simulink model "complementaryAndroidAHRS"  (R2019a)
settings: Solver=FixedStepAuto  StartTime=0.0  StopTime=40  RelTol=1e-3
InitFcn:
  | Ts=0.004
undefined symbols (not defined in the file): DiscIntNeverNeededParam
libraries: simulink_extras x8, androiduilib x6, dspstat3 x3, androidsensorlib x3
PreSaveFcn:
  | set_param(gcs, 'Location',[35 56 895 605])
settings Model: SimulationMode=external  ExtModeTrigDuration=100  Creator=The MathWorks, Inc.  LastModifiedBy=Alireza
settings DataIOCC: LimitDataPoints=on  SaveFormat=Array  ReturnWorkspaceOutputs=off
settings OptimizationCC: LifeSpan=1  MaxStackSize=64
settings DebuggingCC: UnderspecifiedInitializationDetection=Classic  MergeDetectMultiDrivingBlocksExec=none  ParameterPrecisionLossMsg=none  AllowSymbolicDim=off  SFUnexpectedBacktrackingDiag=warning  SFNoUnconditionalDefaultTransitionDiag=warning  SFExecutionAtInitializationDiag=none  ArithmeticOperatorsInVariantConditions=warning
settings HardwareCC: ProdBitPerPointer=32  ProdBitPerSizeT=32  ProdBitPerPtrDiffT=32  ProdLargestAtomicInteger=Long  ProdLargestAtomicFloat=Double  ProdWordSize=32  ProdHWDeviceType=ARM Compatible->ARM Cortex  TargetLargestAtomicInteger=Long  TargetLargestAtomicFloat=Double  TargetEndianess=LittleEndian  TargetHWDeviceType=ARM Compatible->ARM Cortex
settings ModelReferenceCC: PropagateSignalLabelsOutOfModel=off
settings SFSimCC: SimUseLocalCustomCode=off
settings RTWCC: SystemTargetFile=ert.tlc  HardwareBoard=Android Device  TLCOptions="-aInlineSetEventsForThisBaseRateFcn=TLC_FALSE -aSuppressMultiTaskScheduler=TLC_FALSE  -aRateBasedStepFcn=0"  TemplateMakefile=ert_default_tmf  GenerateReport=on  RTWVerbose=off  RTWUseLocalCustomCode=off  Toolchain=Android SDK/NDK Tools  LaunchReport=on
settings CodeAppCC: ForceParamTrailComments=on  OperatorAnnotations=on  MangleLength=10  StateflowObjectComments=on  MATLABSourceComments=on
settings ERTTargetCC: MultiwordLength=2048  ERTCustomFileBanners=off  SupportContinuousTime=on  SupportNonInlinedSFcns=on  RemoveResetFunc=off  SupportVariableSizeSignals=on  ModelStepFunctionPrototypeControlCompliant=off
settings ConfigComp: CovMetricSettings=dw  CovHtmlReporting=on  CovSaveCumulativeToWorkspaceVar=on  CovSaveSingleToWorkspaceVar=on  CovExternalEMLEnable=off  CovSFcnEnable=off

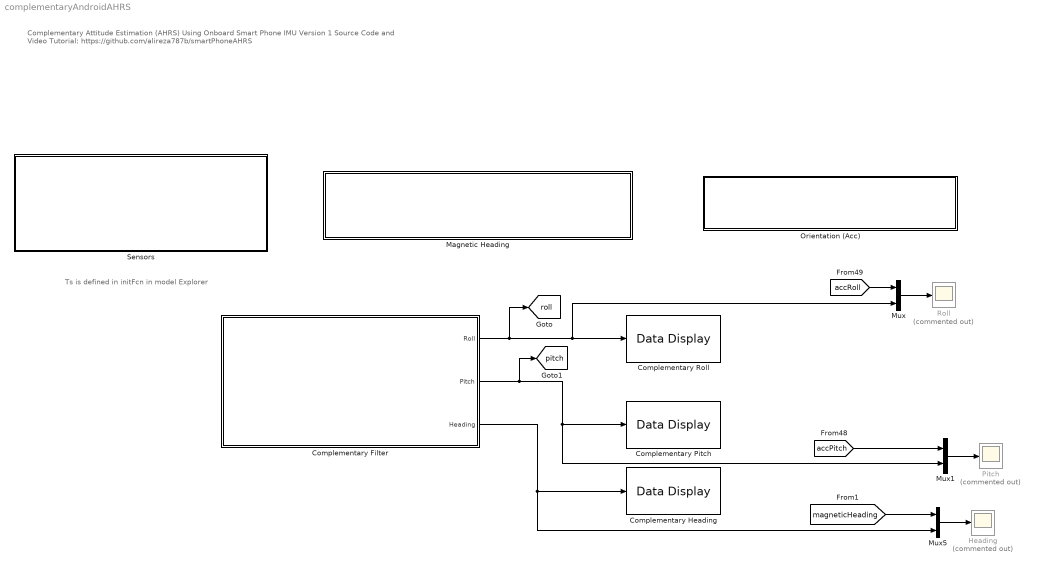
== system complementaryAndroidAHRS ==
  note: Ts is defined in initFcn in model Explorer
  note: Complementary Attitude Estimation (AHRS)
      | Using Onboard Smart Phone IMU Version 1
      | Source Code and Video Tutorial:
      | https://github.com/alireza787b/smartPhoneAHRS
  Complementary Filter : Subsystem
  Complementary Heading : androiduilib/Data Display  DataDisplayId=complementaryAndroidAHRS/Complementary_Heading  Format=Float  Precision=6  SimulateUsing=Code generation  blockPlatform=Android
      settings: SourceProductBaseCode=ANDROID
  Complementary Pitch : androiduilib/Data Display  DataDisplayId=complementaryAndroidAHRS/Complementary_Pitch  Format=Float  Precision=6  SimulateUsing=Code generation  blockPlatform=Android
      settings: SourceProductBaseCode=ANDROID
  Complementary Roll : androiduilib/Data Display  DataDisplayId=complementaryAndroidAHRS/Complementary_Roll  Format=Float  Precision=6  SimulateUsing=Code generation  blockPlatform=Android
      settings: SourceProductBaseCode=ANDROID
  Heading : Scope  Commented=on
  Magnetic Heading : Subsystem
  Mux : Mux  Inputs=2
  Mux1 : Mux  Inputs=2
  Mux5 : Mux  Inputs=2
  Orientation (Acc) : Subsystem
  Pitch : Scope  Commented=on
  Roll : Scope  Commented=on
  Sensors : Subsystem
  tag scope: pitch=global, roll=global
  wires:
  Mux/1 -> Roll/1
  Mux1/1 -> Pitch/1
  Mux5/1 -> Heading/1
  [accPitch] -> Mux1/1
  [accRoll] -> Mux/1
  Complementary Filter/1(Roll) -> Complementary Roll/1, Mux/2, [roll]
  Complementary Filter/2("Pitch ") -> Complementary Pitch/1, Mux1/2, [pitch]
  Complementary Filter/3(Heading) -> Mux5/2, Complementary Heading/1
  [magneticHeading] -> Mux5/1

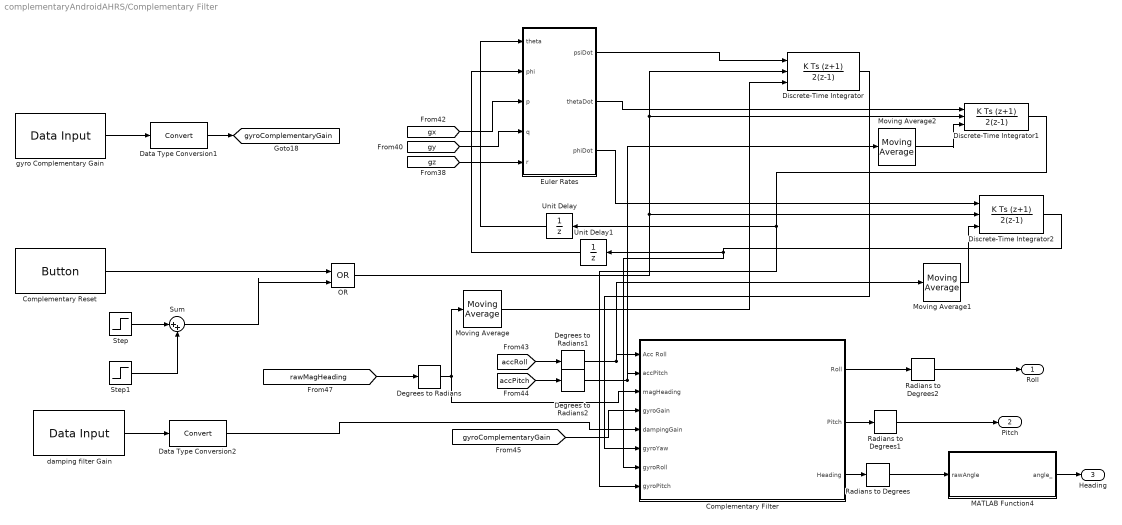
== system complementaryAndroidAHRS/Complementary Filter ==
  Complementary Filter : Subsystem
  Complementary Reset : androiduilib/Button  ButtonState=Not pressed  ButtonId=complementaryAndroidAHRS/Complementary_Filter/Complementary_Reset  State=off  SampleTime=0.1  BlockPlatform=Android
      settings: SourceProductBaseCode=ANDROID
  Data Type Conversion1 : DataTypeConversion
  Data Type Conversion2 : DataTypeConversion
  Degrees to Radians : simulink_extras/Transformations/Degrees to Radians
  Degrees to Radians1 : simulink_extras/Transformations/Degrees to Radians
  Degrees to Radians2 : simulink_extras/Transformations/Degrees to Radians
  Discrete-Time Integrator : DiscreteIntegrator  IntegratorMethod=Integration: Trapezoidal  ExternalReset=either  InitialConditionSource=external  SampleTime=-1  ICPrevOutput=DiscIntNeverNeededParam  ICPrevScaledInput=DiscIntNeverNeededParam
  Discrete-Time Integrator1 : DiscreteIntegrator  IntegratorMethod=Integration: Trapezoidal  ExternalReset=either  InitialConditionSource=external  SampleTime=-1  ICPrevOutput=DiscIntNeverNeededParam  ICPrevScaledInput=DiscIntNeverNeededParam
  Discrete-Time Integrator2 : DiscreteIntegrator  IntegratorMethod=Integration: Trapezoidal  ExternalReset=falling  InitialConditionSource=external  SampleTime=-1  ICPrevOutput=DiscIntNeverNeededParam  ICPrevScaledInput=DiscIntNeverNeededParam
  Euler Rates : Subsystem
  MATLAB Function4 : MATLAB Function  TreatAsAtomicUnit=on
  Moving Average : dspstat3/Moving Average  Method=Sliding window  ForgettingFactorPort=off  SpecifyWindowLength=on  WindowLength=4  ForgettingFactor=0.9  SimulateUsing=Code generation
  Moving Average1 : dspstat3/Moving Average  Method=Sliding window  ForgettingFactorPort=off  SpecifyWindowLength=on  WindowLength=4  ForgettingFactor=0.9  SimulateUsing=Code generation
  Moving Average2 : dspstat3/Moving Average  Method=Sliding window  ForgettingFactorPort=off  SpecifyWindowLength=on  WindowLength=4  ForgettingFactor=0.9  SimulateUsing=Code generation
  OR : Logic  Operator=OR  IconShape=distinctive  AllPortsSameDT=off  OutDataTypeStr=boolean
  Radians to Degrees : simulink_extras/Transformations/Radians to Degrees
  Radians to Degrees1 : simulink_extras/Transformations/Radians to Degrees
  Radians to Degrees2 : simulink_extras/Transformations/Radians to Degrees
  Step : Step  SampleTime=0
  Step1 : Step  Time=2  After=-1  SampleTime=0
  Sum : Sum  Inputs=|++
  Unit Delay : UnitDelay  SampleTime=-1  HasFrameUpgradeWarning=on
  Unit Delay1 : UnitDelay  SampleTime=-1  HasFrameUpgradeWarning=on
  damping filter Gain : androiduilib/Data Input  isCharVector=off  Value=0.9  CharVector=Hello World  OutputDataType=double  maxCharVectorSize=100  DataInputId=complementaryAndroidAHRS/Complementary_Filter/damping_filter_Gain  SampleTime=0.1
      settings: SourceProductBaseCode=ANDROID
  gyro Complementary Gain : androiduilib/Data Input  isCharVector=off  Value=0.78  CharVector=Hello World  OutputDataType=double  maxCharVectorSize=100  DataInputId=complementaryAndroidAHRS/Complementary_Filter/gyro_Complementary_Gain  SampleTime=0.1
      settings: SourceProductBaseCode=ANDROID
  Roll : Outport
  "Pitch " : Outport  Port=2
  Heading : Outport  Port=3
  tag scope: gyroComplementaryGain=global
  wires:
  [gy] -> Euler Rates/4(q)
  Euler Rates/3(phiDot) -> Discrete-Time Integrator2/1
  gyro Complementary Gain/1 -> Data Type Conversion1/1
  Complementary Filter/3(Heading) -> Radians to Degrees/1
  Euler Rates/1(psiDot) -> Discrete-Time Integrator/1
  Discrete-Time Integrator/1 -> Complementary Filter/6(gyroYaw)
  Unit Delay/1 -> Euler Rates/1(theta)
  Complementary Filter/1(Roll) -> Radians to Degrees2/1
  Unit Delay1/1 -> Euler Rates/2(phi)
  Degrees to Radians/1 -> Moving Average/1, Complementary Filter/3(magHeading)
  Discrete-Time Integrator1/1 -> Unit Delay/1, Complementary Filter/8(gyroPitch)
  [accRoll] -> Degrees to Radians1/1
  [gyroComplementaryGain] -> Complementary Filter/4(gyroGain)
  Discrete-Time Integrator2/1 -> Unit Delay1/1, Complementary Filter/7(gyroRoll)
  [rawMagHeading] -> Degrees to Radians/1
  [gx] -> Euler Rates/3(p)
  Euler Rates/2(thetaDot) -> Discrete-Time Integrator1/1
  [gz] -> Euler Rates/5(r)
  [accPitch] -> Degrees to Radians2/1
  Complementary Filter/2(Pitch) -> Radians to Degrees1/1
  Radians to Degrees1/1 -> "Pitch "/1
  Radians to Degrees2/1 -> Roll/1
  Radians to Degrees/1 -> MATLAB Function4/1(rawAngle)
  OR/1 -> Discrete-Time Integrator/2, Discrete-Time Integrator1/2, Discrete-Time Integrator2/2
  Moving Average/1 -> Discrete-Time Integrator/3
  Moving Average1/1 -> Discrete-Time Integrator2/3
  Moving Average2/1 -> Discrete-Time Integrator1/3
  Degrees to Radians1/1 -> Moving Average1/1, Complementary Filter/1(Acc Roll)
  Degrees to Radians2/1 -> Moving Average2/1, Complementary Filter/2(accPitch)
  MATLAB Function4/1(angle_) -> Heading/1
  Data Type Conversion1/1 -> [gyroComplementaryGain]
  Complementary Reset/1 -> OR/1
  Step/1 -> Sum/1
  Step1/1 -> Sum/2
  Sum/1 -> OR/2
  damping filter Gain/1 -> Data Type Conversion2/1
  Data Type Conversion2/1 -> Complementary Filter/5(dampingGain)

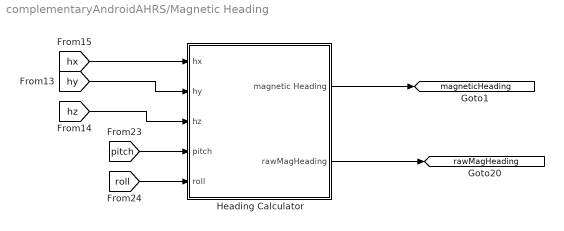
== system complementaryAndroidAHRS/Magnetic Heading ==
  Heading Calculator : Subsystem
  tag scope: magneticHeading=global, rawMagHeading=global
  wires:
  [hz] -> Heading Calculator/3(hz)
  [hy] -> Heading Calculator/2(hy)
  [hx] -> Heading Calculator/1(hx)
  [pitch] -> Heading Calculator/4(pitch)
  [roll] -> Heading Calculator/5(roll)
  Heading Calculator/2(rawMagHeading) -> [rawMagHeading]
  Heading Calculator/1(magnetic Heading) -> [magneticHeading]

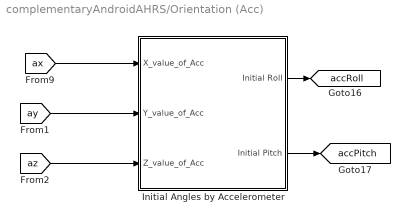
== system complementaryAndroidAHRS/Orientation (Acc) ==
  Initial Angles by Accelerometer : Subsystem
  tag scope: accPitch=global, accRoll=global
  wires:
  [ax] -> Initial Angles by Accelerometer/1(X_value_of_Acc)
  Initial Angles by Accelerometer/2(Initial Pitch) -> [accPitch]
  [ay] -> Initial Angles by Accelerometer/2(Y_value_of_Acc)
  [az] -> Initial Angles by Accelerometer/3(Z_value_of_Acc)
  Initial Angles by Accelerometer/1(Initial Roll) -> [accRoll]

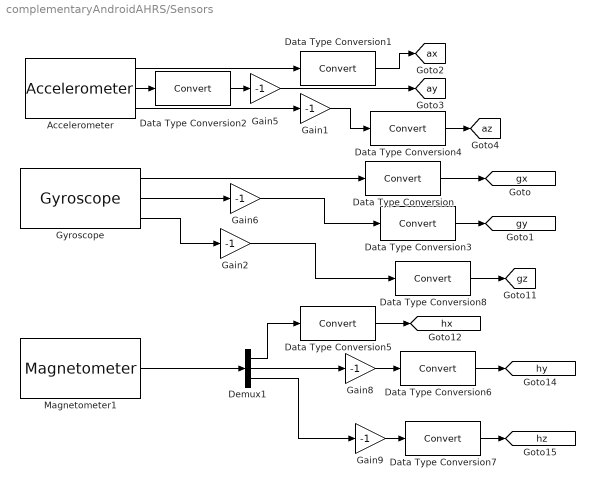
== system complementaryAndroidAHRS/Sensors ==
  Accelerometer : androidsensorlib/Accelerometer  OutputVector=off  SampleTime=Ts  BlockPlatform=Android
      settings: SourceProductBaseCode=ANDROID
  Data Type Conversion{,1..8} (9 alike) : DataTypeConversion
  Demux1 : Demux  Outputs=3
  Gain{1..2,5..6,8..9} (6 alike) : Gain  Gain=-1
  Gyroscope : androidsensorlib/Gyroscope  OutputVector=off  SampleTime=Ts  BlockPlatform=Android
      settings: SourceProductBaseCode=ANDROID
  Magnetometer1 : androidsensorlib/Magnetometer  SampleTime=0.01  SimulateUsing=Code generation
      settings: SourceProductBaseCode=ANDROID
  tag scope: ax=global, ay=global, az=global, gx=global, gy=global, gz=global, hx=global, hy=global, hz=global
  wires:
  Demux1/1 -> Data Type Conversion5/1
  Gain8/1 -> Data Type Conversion6/1
  Data Type Conversion6/1 -> [hy]
  Accelerometer/2 -> Data Type Conversion2/1
  Demux1/3 -> Gain9/1
  Data Type Conversion5/1 -> [hx]
  Gain1/1 -> Data Type Conversion4/1
  Accelerometer/3 -> Gain1/1
  Gyroscope/2 -> Gain6/1
  Data Type Conversion7/1 -> [hz]
  Gain2/1 -> Data Type Conversion8/1
  Data Type Conversion4/1 -> [az]
  Gyroscope/1 -> Data Type Conversion/1
  Data Type Conversion3/1 -> [gy]
  Gain9/1 -> Data Type Conversion7/1
  Gain5/1 -> [ay]
  Data Type Conversion/1 -> [gx]
  Magnetometer1/1 -> Demux1/1
  Gain6/1 -> Data Type Conversion3/1
  Accelerometer/1 -> Data Type Conversion1/1
  Gyroscope/3 -> Gain2/1
  Demux1/2 -> Gain8/1
  Data Type Conversion8/1 -> [gz]
  Data Type Conversion2/1 -> Gain5/1
  Data Type Conversion1/1 -> [ax]

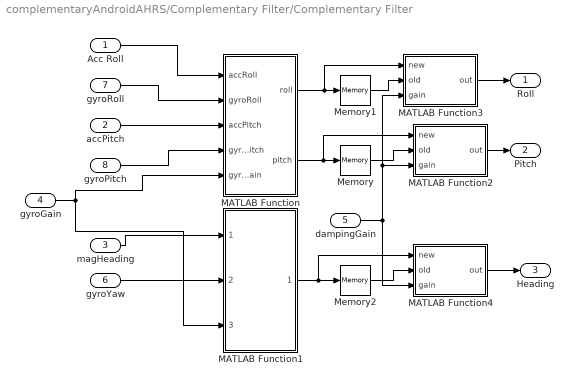
== system complementaryAndroidAHRS/Complementary Filter/Complementary Filter ==
  Acc Roll : Inport
  accPitch : Inport  Port=2
  magHeading : Inport  Port=3
  gyroGain : Inport  Port=4
  dampingGain : Inport  Port=5
  gyroYaw : Inport  Port=6
  gyroRoll : Inport  Port=7
  gyroPitch : Inport  Port=8
  MATLAB Function : MATLAB Function  TreatAsAtomicUnit=on
  MATLAB Function1 : MATLAB Function  TreatAsAtomicUnit=on
  MATLAB Function2 : MATLAB Function  TreatAsAtomicUnit=on
  MATLAB Function3 : MATLAB Function  TreatAsAtomicUnit=on
  MATLAB Function4 : MATLAB Function  TreatAsAtomicUnit=on
  Memory : Memory
  Memory1 : Memory
  Memory2 : Memory
  Roll : Outport
  Pitch : Outport  Port=2
  Heading : Outport  Port=3
  wires:
  MATLAB Function/2(pitch) -> MATLAB Function2/1(new), Memory/1
  gyroPitch/1 -> MATLAB Function/4(gyroPitch)
  accPitch/1 -> MATLAB Function/3(accPitch)
  gyroRoll/1 -> MATLAB Function/2(gyroRoll)
  Acc Roll/1 -> MATLAB Function/1(accRoll)
  gyroYaw/1 -> MATLAB Function1/2(gyroYaw)
  magHeading/1 -> MATLAB Function1/1(magHeading)
  MATLAB Function1/1(heading) -> MATLAB Function4/1(new), Memory2/1
  MATLAB Function/1(roll) -> MATLAB Function3/1(new), Memory1/1
  Memory/1 -> MATLAB Function2/2(old)
  MATLAB Function2/1(out) -> Pitch/1
  MATLAB Function3/1(out) -> Roll/1
  Memory1/1 -> MATLAB Function3/2(old)
  Memory2/1 -> MATLAB Function4/2(old)
  MATLAB Function4/1(out) -> Heading/1
  gyroGain/1 -> MATLAB Function1/3(gyroGainHeading), MATLAB Function/5(gyroGain)
  dampingGain/1 -> MATLAB Function3/3(gain), MATLAB Function2/3(gain), MATLAB Function4/3(gain)

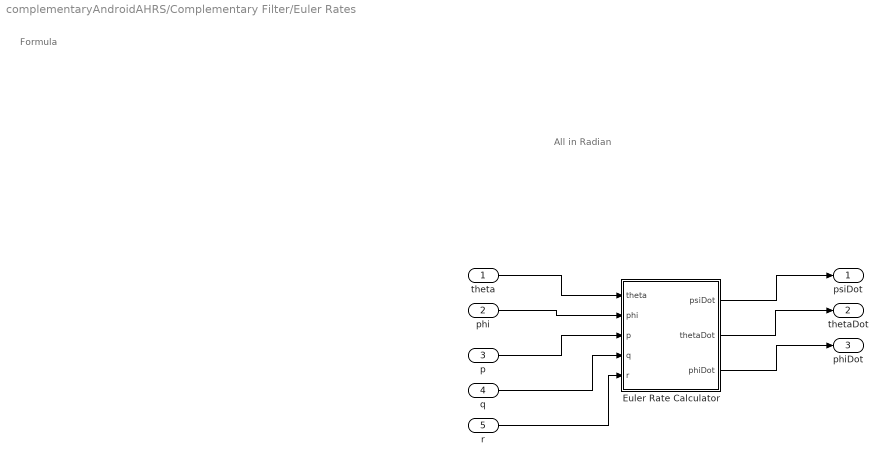
== system complementaryAndroidAHRS/Complementary Filter/Euler Rates ==
  note: All in Radian
  note: Formula
  theta : Inport
  phi : Inport  Port=2
  p : Inport  Port=3
  q : Inport  Port=4
  r : Inport  Port=5
  Euler Rate Calculator : MATLAB Function  TreatAsAtomicUnit=on
  psiDot : Outport
  thetaDot : Outport  Port=2
  phiDot : Outport  Port=3
  wires:
  phi/1 -> Euler Rate Calculator/2(phi)
  theta/1 -> Euler Rate Calculator/1(theta)
  p/1 -> Euler Rate Calculator/3(p)
  q/1 -> Euler Rate Calculator/4(q)
  r/1 -> Euler Rate Calculator/5(r)
  Euler Rate Calculator/1(psiDot) -> psiDot/1
  Euler Rate Calculator/2(thetaDot) -> thetaDot/1
  Euler Rate Calculator/3(phiDot) -> phiDot/1

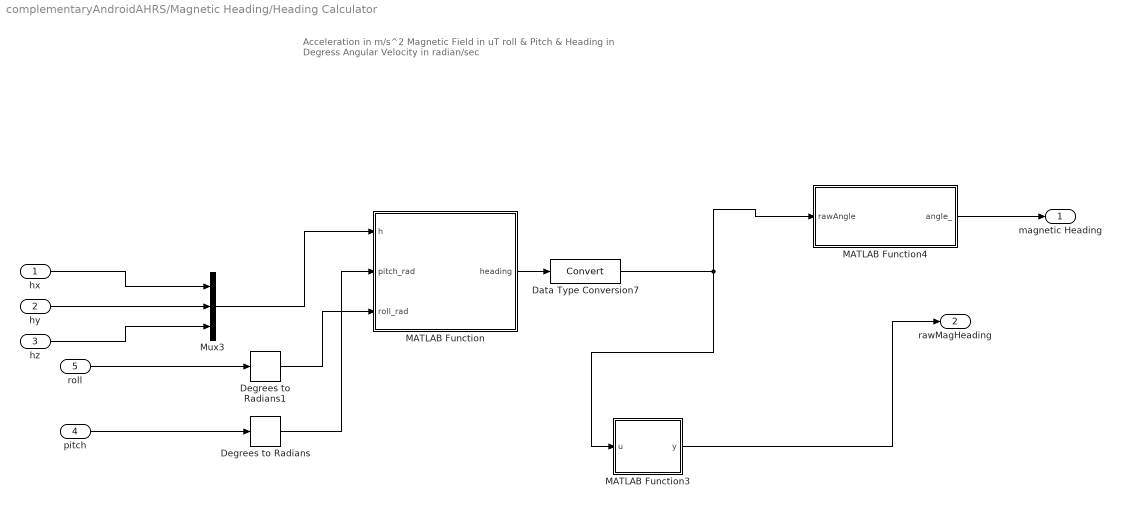
== system complementaryAndroidAHRS/Magnetic Heading/Heading Calculator ==
  note: Acceleration in m/s^2
      | Magnetic Field in uT
      | roll & Pitch & Heading in Degress
      | Angular Velocity in radian/sec
  hx : Inport
  hy : Inport  Port=2
  hz : Inport  Port=3
  pitch : Inport  Port=4
  roll : Inport  Port=5
  Data Type Conversion7 : DataTypeConversion
  Degrees to Radians : simulink_extras/Transformations/Degrees to Radians
  Degrees to Radians1 : simulink_extras/Transformations/Degrees to Radians
  MATLAB Function : MATLAB Function  TreatAsAtomicUnit=on
  MATLAB Function3 : MATLAB Function  TreatAsAtomicUnit=on
  MATLAB Function4 : MATLAB Function  TreatAsAtomicUnit=on
  Mux3 : Mux  Inputs=3
  magnetic Heading : Outport
  rawMagHeading : Outport  Port=2
  wires:
  hy/1 -> Mux3/2
  MATLAB Function3/1(y) -> rawMagHeading/1
  MATLAB Function/1(heading) -> Data Type Conversion7/1
  roll/1 -> Degrees to Radians1/1
  Data Type Conversion7/1 -> MATLAB Function3/1(u), MATLAB Function4/1(rawAngle)
  MATLAB Function4/1(angle_) -> magnetic Heading/1
  Mux3/1 -> MATLAB Function/1(h)
  Degrees to Radians/1 -> MATLAB Function/2(pitch_rad)
  Degrees to Radians1/1 -> MATLAB Function/3(roll_rad)
  hz/1 -> Mux3/3
  pitch/1 -> Degrees to Radians/1
  hx/1 -> Mux3/1

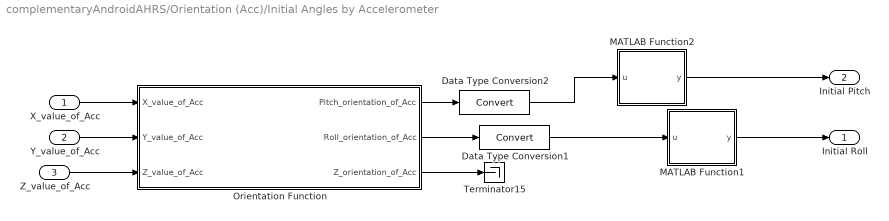
== system complementaryAndroidAHRS/Orientation (Acc)/Initial Angles by Accelerometer ==
  X_value_of_Acc : Inport
  Y_value_of_Acc : Inport  Port=2
  Z_value_of_Acc : Inport  Port=3
  Data Type Conversion1 : DataTypeConversion
  Data Type Conversion2 : DataTypeConversion
  MATLAB Function1 : MATLAB Function  TreatAsAtomicUnit=on
  MATLAB Function2 : MATLAB Function  TreatAsAtomicUnit=on
  Orientation Function : MATLAB Function  TreatAsAtomicUnit=on
  Terminator15 : Terminator
  Initial Roll : Outport
  Initial Pitch : Outport  Port=2
  wires:
  Orientation Function/2(Roll_orientation_of_Acc) -> Data Type Conversion1/1
  Data Type Conversion1/1 -> MATLAB Function1/1(u)
  X_value_of_Acc/1 -> Orientation Function/1(X_value_of_Acc)
  Y_value_of_Acc/1 -> Orientation Function/2(Y_value_of_Acc)
  Orientation Function/1(Pitch_orientation_of_Acc) -> Data Type Conversion2/1
  MATLAB Function2/1(y) -> Initial Pitch/1
  Data Type Conversion2/1 -> MATLAB Function2/1(u)
  Orientation Function/3(Z_orientation_of_Acc) -> Terminator15/1
  Z_value_of_Acc/1 -> Orientation Function/3(Z_value_of_Acc)
  MATLAB Function1/1(y) -> Initial Roll/1

== matlab function complementaryAndroidAHRS/Orientation (Acc)/Initial Angles by Accelerometer/MATLAB Function2 ==
  data: u input; y output
function y = fcn(u)

if(isnan(u))
y=0;
else
y=u;
end

== matlab function complementaryAndroidAHRS/Orientation (Acc)/Initial Angles by Accelerometer/Orientation Function ==
  data: X_value_of_Acc input; Pitch_orientation_of_Acc output; Roll_orientation_of_Acc output; Z_orientation_of_Acc output; Y_value_of_Acc input; Z_value_of_Acc input
% Computing orientation of tri-axial acclerometer data from IMU 
% Author: RM van Rensburg
% Date: 26-04-2015
% Version: 1.0,tested on Matlab R2015a

function [Pitch_orientation_of_Acc,...
          Roll_orientation_of_Acc,...
          Z_orientation_of_Acc]...
          = OrientationFcn(X_value_of_Acc,Y_value_of_Acc,Z_value_of_Acc)
     
      
% Using x and y from accelerometer (g-forces), calculate x and y angles
% Data directly obtained from IMU
% Using the following formulae
% Ax = arctan{X/sqrt(Y*Y + Z*Z)}
% Ay = arctan{Y/sqrt(X*X + Z*Z)}

% Computing the X*X, Y*Y, Z*Z
X2 = power(X_value_of_Acc,2);
Y2 = power(Y_value_of_Acc,2);
Z2 = power(Z_value_of_Acc,2);

% x-axis angle
result = sqrt(Y2 + Z2);
result = X_value_of_Acc / result;
x_angle_rad = atan(result);
Pitch_orientation_of_Acc = (x_angle_rad * 180) / pi;

% y-axis angle
result = sqrt(X2 + Z2);
result = Y_value_of_Acc / result;
y_angle_rad = atan(result);
Roll_orientation_of_Acc = -(y_angle_rad * 180) / pi;

% z-axis angle
result = sqrt(Y2 + X2);
result = Z_value_of_Acc / result;
z_angle_rad = atan(result);
Z_orientation_of_Acc = (z_angle_rad * 180) / pi;

end

== matlab function complementaryAndroidAHRS/Orientation (Acc)/Initial Angles by Accelerometer/MATLAB Function1 ==
  data: u input; y output
function y = fcn(u)

if(isnan(u))
y=0;
else
y=u;
end

== matlab function complementaryAndroidAHRS/Complementary Filter/MATLAB Function4 ==
  data: rawAngle input; angle_ output
function angle_ = constrainerHeading(rawAngle)
angle_ = rawAngle;
    if rawAngle > 360 ;
        angle_ = rawAngle - 360;
    elseif angle_ < 0;
       angle_ =  rawAngle + 360;
    end
end

== matlab function complementaryAndroidAHRS/Complementary Filter/Euler Rates/Euler Rate Calculator ==
  data: theta input; psiDot output; phi input; p input; q input; r input; thetaDot output; phiDot output
function [psiDot,thetaDot,phiDot] = fcn(theta,phi,p,q,r)

psiDot =  sin(phi)/cos(theta)*q + cos(phi)/cos(theta)*r;
thetaDot = cos(phi)*q - sin(phi)*r;
phiDot = p + sin(phi)*tan(theta)*q + cos(phi)*tan(theta)*r;
end

== matlab function complementaryAndroidAHRS/Complementary Filter/Complementary Filter/MATLAB Function ==
  data: accRoll input; roll output; gyroRoll input; accPitch input; gyroPitch input; gyroGain input; pitch output
function [roll,pitch] = fcn(accRoll,gyroRoll,accPitch,gyroPitch,gyroGain)
roll = gyroGain * gyroRoll + (1-gyroGain)*accRoll;
pitch = gyroGain * gyroPitch + (1-gyroGain)*accPitch;

end

== matlab function complementaryAndroidAHRS/Complementary Filter/Complementary Filter/MATLAB Function1 ==
  data: magHeading input; heading output; gyroYaw input; gyroGainHeading input
function heading  = headingCalc(magHeading,gyroYaw,gyroGainHeading)
heading = gyroGainHeading * gyroYaw + (1-gyroGainHeading)*magHeading;
end

== matlab function complementaryAndroidAHRS/Complementary Filter/Complementary Filter/MATLAB Function2 ==
  data: new input; out output; old input; gain input
function out = damper(new,old,gain)
out = gain * old + (1-gain)*new;
end

== matlab function complementaryAndroidAHRS/Complementary Filter/Complementary Filter/MATLAB Function3 ==
  data: new input; out output; old input; gain input
function out = damper(new,old,gain)
out = gain * old + (1-gain)*new;
end

== matlab function complementaryAndroidAHRS/Complementary Filter/Complementary Filter/MATLAB Function4 ==
  data: new input; out output; old input; gain input
function out = damper(new,old,gain)
out = gain * old + (1-gain)*new;
end

== matlab function complementaryAndroidAHRS/Magnetic Heading/Heading Calculator/MATLAB Function ==
  data: heading output; h input; pitch_rad input; roll_rad input
function heading  = mag2Heading(h,pitch_rad,roll_rad)
 h = normalize(h,'norm');
   
    heading_rad = atan2(h(3) * sin(roll_rad) - h(2) * cos(roll_rad), h(1) * cos(pitch_rad) + h(2) * sin(pitch_rad) * sin(roll_rad) + h(3) * sin(pitch_rad) * cos(roll_rad));
    heading = rad2deg(heading_rad);

== matlab function complementaryAndroidAHRS/Magnetic Heading/Heading Calculator/MATLAB Function3 ==
  data: u input; y output
function y = fcn(u)

if(isnan(u))
y=0;
else
y=u;
end

== matlab function complementaryAndroidAHRS/Magnetic Heading/Heading Calculator/MATLAB Function4 ==
  data: rawAngle input; angle_ output
function angle_ = constrainerHeading(rawAngle)
angle_ = rawAngle;
    if rawAngle > 360 ;
        angle_ = rawAngle - 360;
    elseif angle_ < 0;
       angle_ =  rawAngle + 360;
    end
end
